simulink model "ctrl_TT_ad_ctrl_cpp_ros_feedback"  (R2022b)
settings: Solver=FixedStepAuto  StartTime=0.0  StopTime=Tf  FixedStep=0.05  RelTol=1e-3
StopFcn:
  | save('testdata')
values from neighbouring files (symbols this model uses):
  adap = 1    [testdata.mat]
  Ba_0 = [0 0 0 0 0 0]    [testdata.mat]
  Bb = 4418825.3321    [testdata.mat]
  Bv_0 = [-5.14444 0 0 0 0 0]    [testdata.mat]
  Bx_0 = [70.34790039 -18.70597267 -370.8000183 0 0 0]    [testdata.mat]
  Cp = [-70.34790039 18.70597267 -370.8000183 -33.25566673 18.72042656 -369.9571533 3.8263092 17.99342728 -368.5174255 40.77630615 14.78142262 -366.2670288 ... (183 elements, 3x61)]    [testdata.mat]    (also in tester.m = [Cpx'; Cpy'; Cpz'])
  Cp_prime = [4.4510680392 0.0017344668 0.1011438 4.44985762706 -0.08575700726 0.1715736104 4.43452754992 -0.37550053768 0.2668049284 4.4276356638 -0.45576590634 0.3213246444 ... (183 elements, 3x61)]    [testdata.mat]
  d = 250    [testdata.mat]
  dA_BP1 = [0.00388591051125 0.00354364911083 0.00553040741788 0.00502167988714 0.0078585088908 0.00748424955325 0.0119232766011 0.0109054787122 0.0168329706434 0.016985509009 0.0156802934897 0.014556760782 ... (616 elements, 616x1)]    [testdata.mat]
  dA_BP2 = [0.00388594063171 0.00354357191533 0.00553040491113 0.00502170939051 0.00785855989083 0.00748435285791 0.0119232653011 0.0109054419481 0.0168329955973 0.0169854794658 0.015680230324 0.0145567225609 ... (616 elements, 616x1)]    [testdata.mat]
  dA_Hull = [0.896301676511 0.898896720864 0.884294141897 0.886832830172 0.870887902011 0.873360353662 0.856223658523 0.858613244346 0.840314828191 0.842595287849 0.823129385532 0.8253007603 ... (2914 elements, 2914x1)]    [testdata.mat]
  dA_PH = [0.00917454029683 0.00917454029683 0.00646521761836 0.00644666811643 0.011728531678 0.0107683420972 0.0165186720105 0.0100399866209 0.0121147162203 0.00917369783051 0.00917369783051 0.00646462373197 ... (550 elements, 550x1)]    [testdata.mat]
  dA_Sail = [0.08073747293 0.0655437895785 0.0678199581962 0.211496702297 0.185444652254 0.10949647106 0.0763960001413 0.0735864235671 0.0440728222699 0.281106392154 0.32735958292 0.104041938486 ... (564 elements, 564x1)]    [testdata.mat]
  dA_SProot = [0.0225345452169 0.0247277274893 0.0225345452169 0.0480467976325 0.0166447079844 0.0410754287554 0.0247277274893 0.0480467976325 0.0468898715351 0.0839833312794 0.0166447079844 0.0255016718 ... (904 elements, 904x1)]    [testdata.mat]
  dA_X1a = [0.0149621011817 0.0166706156701 0.0341149781095 0.0355915100668 0.0512235531199 0.0489176133683 0.0604458424392 0.0503279152264 0.0577124835488 0.0401555322121 0.044833653096 0.0251568218541 ... (200 elements, 200x1)]    [testdata.mat]
  dA_X1b = [0.0149621011817 0.0166706156701 0.0341149781095 0.0355915100668 0.0512235531199 0.0489176133683 0.0604458424392 0.0503279152264 0.0577124835488 0.0401555322121 0.044833653096 0.0251568218541 ... (200 elements, 200x1)]    [testdata.mat]
  dA_X2a = [0.0149620639393 0.0166705502855 0.0341150948266 0.0355913495849 0.051223110376 0.0489180393921 0.0604458270347 0.0503275686692 0.0577128112225 0.0401556683139 0.0448334591683 0.0251566482124 ... (200 elements, 200x1)]    [testdata.mat]
  dA_X2b = [0.0149620639393 0.0166705502855 0.0341150948266 0.0355913495849 0.051223110376 0.0489180393921 0.0604458270347 0.0503275686692 0.0577128112225 0.0401556683139 0.0448334591683 0.0251566482124 ... (200 elements, 200x1)]    [testdata.mat]
  dA_X3a = [0.0149621011817 0.0166706156701 0.0341149781095 0.0355915100668 0.0512235531199 0.0489176133683 0.0604458424392 0.0503279152264 0.0577124835488 0.0401555322121 0.044833653096 0.0251568218541 ... (200 elements, 200x1)]    [testdata.mat]
  dA_X3b = [0.0149621011817 0.0166706156701 0.0341149781095 0.0355915100668 0.0512235531199 0.0489176133683 0.0604458424392 0.0503279152264 0.0577124835488 0.0401555322121 0.044833653096 0.0251568218541 ... (200 elements, 200x1)]    [testdata.mat]
  dA_X4a = [0.0149621011817 0.0166706156701 0.0341149781095 0.0355915100668 0.0512235531199 0.0489176133683 0.0604458424392 0.0503279152264 0.0577124835488 0.0401555322121 0.044833653096 0.0251568218541 ... (200 elements, 200x1)]    [testdata.mat]
  dA_X4b = [0.0149621011817 0.0166706156701 0.0341149781095 0.0355915100668 0.0512235531199 0.0489176133683 0.0604458424392 0.0503279152264 0.0577124835488 0.0401555322121 0.044833653096 0.0251568218541 ... (200 elements, 200x1)]    [testdata.mat]
  Ixx = 52300000    [testdata.mat]
  Ixy = 0    [testdata.mat]
  Ixz = 0    [testdata.mat]
  Iyy = 1375000000    [testdata.mat]
  Iyz = 0    [testdata.mat]
  Izz = 1367000000    [testdata.mat]
  Kp = 0.1    [testdata.mat]
  L1 =     [testdata.mat]
  Mb = 4418825.3321    [testdata.mat]
  n_BP1 = [-0.7747315 -0.03638153 -0.4095958 0 -0.1221389 0 -0.01670914 0 0.005209626 0 0.03404154 0 ... (1848 elements, 616x3)]    [testdata.mat]
  n_BP2 = [-0.774731517 -0.0363815315 -0.409595788 0 -0.122138903 0 -0.0167091396 0 0.00520962616 0 0.0340415388 0 ... (1848 elements, 616x3)]    [testdata.mat]
  n_Hull = [-3.334458e-05 -1.700098e-14 -3.354233e-05 -1.686235e-14 -3.289162e-05 -1.685701e-14 -3.291391e-05 -1.698144e-14 -3.338145e-05 -1.688959e-14 -3.29289e-05 -1.682536e-14 ... (8742 elements, 2914x3)]    [testdata.mat]
  n_PH = [0 0 0.01711651 0.01711627 0.2676807 0.2676804 0.7675173 0.7675174 0.9857236 0 0 0.01711456 ... (1650 elements, 550x3)]    [testdata.mat]
  n_Sail = [-0.05126832 -0.05168081 -0.0485872 -0.03288998 -0.03203588 -0.04435105 -0.04335441 -0.04419429 -0.05169604 0.01094904 0.01649325 -0.03825178 ... (1692 elements, 564x3)]    [testdata.mat]
  n_SProot = [-0.7837688 -0.7969784 -0.7837688 -0.79448 -0.280412 -0.3378876 -0.7969784 -0.79448 -0.7910827 -0.3483897 -0.280412 -0.2790298 ... (2712 elements, 904x3)]    [testdata.mat]
  n_X2a = [-0.283297986 -0.283136904 -0.283195704 -0.28313759 -0.2831586 -0.283137113 -0.28313911 -0.283136606 -0.283121586 -0.283136815 -0.283108413 -0.283138901 ... (600 elements, 200x3)]    [testdata.mat]
  n_X2b = [-0.283297986 -0.283136904 -0.283195704 -0.28313759 -0.2831586 -0.283137113 -0.28313911 -0.283136606 -0.283121586 -0.283136815 -0.283108413 -0.283138901 ... (600 elements, 200x3)]    [testdata.mat]
  n_X3a = [-0.283298 -0.2831369 -0.2831957 -0.2831376 -0.2831586 -0.2831371 -0.2831391 -0.2831366 -0.2831216 -0.2831368 -0.2831084 -0.2831389 ... (600 elements, 200x3)]    [testdata.mat]
  n_X4a = [-0.283298 -0.2831369 -0.2831957 -0.2831376 -0.2831586 -0.2831371 -0.2831391 -0.2831366 -0.2831216 -0.2831368 -0.2831084 -0.2831389 ... (600 elements, 200x3)]    [testdata.mat]
  n_X4b = [-0.283298 -0.2831369 -0.2831957 -0.2831376 -0.2831586 -0.2831371 -0.2831391 -0.2831366 -0.2831216 -0.2831368 -0.2831084 -0.2831389 ... (600 elements, 200x3)]    [testdata.mat]
  nt_BP1 = 616    [testdata.mat]
  nt_BP2 = 616    [testdata.mat]
  nt_Hull = 2914    [testdata.mat]
  nt_PH = 550    [testdata.mat]
  nt_Sail = 564    [testdata.mat]
  nt_SProot = 904    [testdata.mat]
  nt_X1a = 200    [testdata.mat]
  nt_X1b = 200    [testdata.mat]
  nt_X2a = 200    [testdata.mat]
  nt_X2b = 200    [testdata.mat]
  nt_X3a = 200    [testdata.mat]
  nt_X3b = 200    [testdata.mat]
  nt_X4a = 200    [testdata.mat]
  nt_X4b = 200    [testdata.mat]
  Seastate = 0    [testdata.mat]
  Tf = 500    [testdata.mat]    (also in tester.m)
  Ts = 0.05    [testdata.mat]
  vt1_BP1 = [-11.0524049722 -10.9924120522 -10.9924120522 -10.8819663922 -10.8819663922 -10.7297166322 -10.7297166322 -10.5070632922 -10.5070632922 -10.1807245522 -10.1807245522 -9.8815181122 ... (1848 elements, 616x3)]    [testdata.mat]
  vt1_BP2 = [-11.0524048318 -10.9924111396 -10.9924111396 -10.8819658306 -10.8819658306 -10.7297157898 -10.7297157898 -10.5070637134 -10.5070637134 -10.1807238502 -10.1807238502 -9.8815188844 ... (1848 elements, 616x3)]    [testdata.mat]
  vt1_Hull = [3.5122487678 3.7304022878 5.2621803278 5.4863499878 6.9866994878 7.2167238278 8.6832650078 8.9189474678 10.3493567078 10.5904445678 11.9823842078 12.2286247478 ... (8742 elements, 2914x3)]    [testdata.mat]
  vt1_PH = [37.3342788278 37.3342788278 37.4268866678 37.4268866678 37.5892452278 37.5892452278 37.7549453078 37.7549453078 37.8074619278 37.3342788278 37.3342788278 37.4268866678 ... (1650 elements, 550x3)]    [testdata.mat]
  vt1_Sail = [-12.4909433722 -12.1578443722 -12.0399645322 -11.2138368922 -10.6240515922 -11.5111900522 -11.9364967522 -11.6561249722 -12.4909433722 -7.5732648922 -6.8453119522 -11.1890071522 ... (1692 elements, 564x3)]    [testdata.mat]
  vt1_SProot = [29.2099766678 29.1371231078 29.0494854278 29.2099766678 29.2862630078 29.4526510478 29.0494854278 29.1261368078 29.3369263478 29.5706712878 29.0494854278 29.3857364078 ... (2712 elements, 904x3)]    [testdata.mat]
  vt1_X1a = [29.3961751478 29.4776282078 29.4776282078 29.7060309278 29.7060309278 30.0693861278 30.0693861278 30.5458756478 30.5458756478 31.0830460478 31.0830460478 31.6023926678 ... (600 elements, 200x3)]    [testdata.mat]
  vt1_X1b = [29.6638337078 29.6638337078 29.9620713878 29.9620713878 30.3181187678 30.3181187678 30.7116389078 30.7116389078 31.1104380878 31.1104380878 31.4810519678 31.4810519678 ... (600 elements, 200x3)]    [testdata.mat]
  vt1_X2a = [29.3961767624 29.4776272952 29.4776272952 29.7060326828 29.7060326828 30.0693842324 30.0693842324 30.5458736822 30.5458736822 31.083047171 31.083047171 31.6023916148 ... (600 elements, 200x3)]    [testdata.mat]
  vt1_X2b = [29.6638345502 29.6638345502 29.9620708964 29.9620708964 30.3181168022 30.3181168022 30.7116409436 30.7116409436 31.1104372454 31.1104372454 31.4810526698 31.4810526698 ... (600 elements, 200x3)]    [testdata.mat]
  vt1_X3a = [29.3961751478 29.4776282078 29.4776282078 29.7060309278 29.7060309278 30.0693861278 30.0693861278 30.5458756478 30.5458756478 31.0830460478 31.0830460478 31.6023926678 ... (600 elements, 200x3)]    [testdata.mat]
  vt1_X3b = [29.6638337078 29.6638337078 29.9620713878 29.9620713878 30.3181187678 30.3181187678 30.7116389078 30.7116389078 31.1104380878 31.1104380878 31.4810519678 31.4810519678 ... (600 elements, 200x3)]    [testdata.mat]
  vt1_X4a = [29.6638337078 29.6638337078 29.9620713878 29.9620713878 30.3181187678 30.3181187678 30.7116389078 30.7116389078 31.1104380878 31.1104380878 31.4810519678 31.4810519678 ... (600 elements, 200x3)]    [testdata.mat]
  vt1_X4b = [29.3961751478 29.4776282078 29.4776282078 29.7060309278 29.7060309278 30.0693861278 30.0693861278 30.5458756478 30.5458756478 31.0830460478 31.0830460478 31.6023926678 ... (600 elements, 200x3)]    [testdata.mat]
  vt2_BP1 = [-10.9924120522 -10.9494777322 -10.8819663922 -10.8505308322 -10.7297166322 -10.7112259522 -10.5070632922 -10.4997203722 -10.1807245522 -10.1757543922 -9.8815181122 -9.8813004922 ... (1848 elements, 616x3)]    [testdata.mat]
  vt2_BP2 = [-11.0294626294 -11.0294626294 -10.9494786448 -10.9494786448 -10.8505316746 -10.8505316746 -10.7112256012 -10.7112256012 -10.499720302 -10.499720302 -10.1757550942 -10.1757550942 ... (1848 elements, 616x3)]    [testdata.mat]
  vt2_Hull = [1.9517168078 1.9517168078 3.7304022878 3.7304022878 5.4863499878 5.4863499878 7.2167238278 7.2167238278 8.9189474678 8.9189474678 10.5904445678 10.5904445678 ... (8742 elements, 2914x3)]    [testdata.mat]
  vt2_PH = [37.2028433678 37.2028433678 37.3342788278 37.4268866678 37.4268866678 37.5892452278 37.5892452278 37.7549453078 37.7549453078 37.2028433678 37.2028433678 37.3342788278 ... (1650 elements, 550x3)]    [testdata.mat]
  vt2_Sail = [-12.0399645322 -12.0399645322 -11.9364967522 -10.7084881522 -10.7084881522 -12.0399645322 -12.0399645322 -11.9364967522 -12.3734566522 -7.7110323922 -7.7110323922 -11.6561249722 ... (1692 elements, 564x3)]    [testdata.mat]
  vt2_SProot = [29.0494854278 29.0494854278 29.2099766678 29.1261368078 29.0494854278 29.1371231078 29.1371231078 29.2099766678 29.1261368078 29.2099766678 29.2862630078 29.2862630078 ... (2712 elements, 904x3)]    [testdata.mat]
  vt2_X1a = [29.4776282078 29.9620713878 29.7060309278 30.3181187678 30.0693861278 30.7116389078 30.5458756478 31.1104380878 31.0830460478 31.4810519678 31.6023926678 31.7970362078 ... (600 elements, 200x3)]    [testdata.mat]
  vt2_X1b = [29.4776282078 29.9620713878 29.7060309278 30.3181187678 30.0693861278 30.7116389078 30.5458756478 31.1104380878 31.0830460478 31.4810519678 31.6023926678 31.7970362078 ... (600 elements, 200x3)]    [testdata.mat]
  vt2_X2a = [29.6638345502 29.6638345502 29.9620708964 29.9620708964 30.3181168022 30.3181168022 30.7116409436 30.7116409436 31.1104372454 31.1104372454 31.4810526698 31.4810526698 ... (600 elements, 200x3)]    [testdata.mat]
  vt2_X2b = [29.3961767624 29.4776272952 29.4776272952 29.7060326828 29.7060326828 30.0693842324 30.0693842324 30.5458736822 30.5458736822 31.083047171 31.083047171 31.6023916148 ... (600 elements, 200x3)]    [testdata.mat]
  vt2_X3a = [29.4776282078 29.9620713878 29.7060309278 30.3181187678 30.0693861278 30.7116389078 30.5458756478 31.1104380878 31.0830460478 31.4810519678 31.6023926678 31.7970362078 ... (600 elements, 200x3)]    [testdata.mat]
  vt2_X3b = [29.4776282078 29.9620713878 29.7060309278 30.3181187678 30.0693861278 30.7116389078 30.5458756478 31.1104380878 31.0830460478 31.4810519678 31.6023926678 31.7970362078 ... (600 elements, 200x3)]    [testdata.mat]
  vt2_X4a = [29.4776282078 29.9620713878 29.7060309278 30.3181187678 30.0693861278 30.7116389078 30.5458756478 31.1104380878 31.0830460478 31.4810519678 31.6023926678 31.7970362078 ... (600 elements, 200x3)]    [testdata.mat]
  vt2_X4b = [29.4776282078 29.9620713878 29.7060309278 30.3181187678 30.0693861278 30.7116389078 30.5458756478 31.1104380878 31.0830460478 31.4810519678 31.6023926678 31.7970362078 ... (600 elements, 200x3)]    [testdata.mat]
  vt3_BP1 = [-11.0294636122 -11.0294636122 -10.9494777322 -10.9494777322 -10.8505308322 -10.8505308322 -10.7112259522 -10.7112259522 -10.4997203722 -10.4997203722 -10.1757543922 -10.1757543922 ... (1848 elements, 616x3)]    [testdata.mat]
  vt3_BP2 = [-10.9924111396 -10.9494786448 -10.8819658306 -10.8505316746 -10.7297157898 -10.7112256012 -10.5070637134 -10.499720302 -10.1807238502 -10.1757550942 -9.8815188844 -9.8813013346 ... (1848 elements, 616x3)]    [testdata.mat]
  vt3_Hull = [1.7397198278 3.5122487678 3.5122487678 5.2621803278 5.2621803278 6.9866994878 6.9866994878 8.6832650078 8.6832650078 10.3493567078 10.3493567078 11.9823842078 ... (8742 elements, 2914x3)]    [testdata.mat]
  vt3_PH = [37.2028433678 37.3342788278 37.3342788278 37.3342788278 37.4268866678 37.4268866678 37.5892452278 37.5892452278 37.7549453078 37.2028433678 37.3342788278 37.3342788278 ... (1650 elements, 550x3)]    [testdata.mat]
  vt3_Sail = [-12.3734566522 -12.4909433722 -12.3734566522 -11.5111900522 -11.2138368922 -11.7698559922 -11.5111900522 -11.5111900522 -12.1578443722 -8.3109054322 -7.5732648922 -11.5111900522 ... (1692 elements, 564x3)]    [testdata.mat]
  vt3_SProot = [29.1261368078 29.2099766678 29.1261368078 29.3369263478 29.1371231078 29.2099766678 29.2099766678 29.3369263478 29.2548344678 29.3369263478 29.1371231078 29.1371231078 ... (2712 elements, 904x3)]    [testdata.mat]
  vt3_X1a = [29.6638337078 29.6638337078 29.9620713878 29.9620713878 30.3181187678 30.3181187678 30.7116389078 30.7116389078 31.1104380878 31.1104380878 31.4810519678 31.4810519678 ... (600 elements, 200x3)]    [testdata.mat]
  vt3_X1b = [29.3961751478 29.4776282078 29.4776282078 29.7060309278 29.7060309278 30.0693861278 30.0693861278 30.5458756478 30.5458756478 31.0830460478 31.0830460478 31.6023926678 ... (600 elements, 200x3)]    [testdata.mat]
  vt3_X2a = [29.4776272952 29.9620708964 29.7060326828 30.3181168022 30.0693842324 30.7116409436 30.5458736822 31.1104372454 31.083047171 31.4810526698 31.6023916148 31.7970343826 ... (600 elements, 200x3)]    [testdata.mat]
  vt3_X2b = [29.4776272952 29.9620708964 29.7060326828 30.3181168022 30.0693842324 30.7116409436 30.5458736822 31.1104372454 31.083047171 31.4810526698 31.6023916148 31.7970343826 ... (600 elements, 200x3)]    [testdata.mat]
  vt3_X3a = [29.6638337078 29.6638337078 29.9620713878 29.9620713878 30.3181187678 30.3181187678 30.7116389078 30.7116389078 31.1104380878 31.1104380878 31.4810519678 31.4810519678 ... (600 elements, 200x3)]    [testdata.mat]
  vt3_X3b = [29.3961751478 29.4776282078 29.4776282078 29.7060309278 29.7060309278 30.0693861278 30.0693861278 30.5458756478 30.5458756478 31.0830460478 31.0830460478 31.6023926678 ... (600 elements, 200x3)]    [testdata.mat]
  vt3_X4a = [29.3961751478 29.4776282078 29.4776282078 29.7060309278 29.7060309278 30.0693861278 30.0693861278 30.5458756478 30.5458756478 31.0830460478 31.0830460478 31.6023926678 ... (600 elements, 200x3)]    [testdata.mat]
  vt3_X4b = [29.6638337078 29.6638337078 29.9620713878 29.9620713878 30.3181187678 30.3181187678 30.7116389078 30.7116389078 31.1104380878 31.1104380878 31.4810519678 31.4810519678 ... (600 elements, 200x3)]    [testdata.mat]
  Xb = 0    [testdata.mat]
  Xcg = [32.3287332922 0 0]    [testdata.mat]
  Xg = 0    [testdata.mat]
  Yb = 0    [testdata.mat]
  Yg = 0    [testdata.mat]
  Zb = 0.4406    [testdata.mat]
  Zg = 0    [testdata.mat]
libraries: robotlib x54, simulink x8, sharedtransform x2, dspmathops x2
(part 5 of 9)

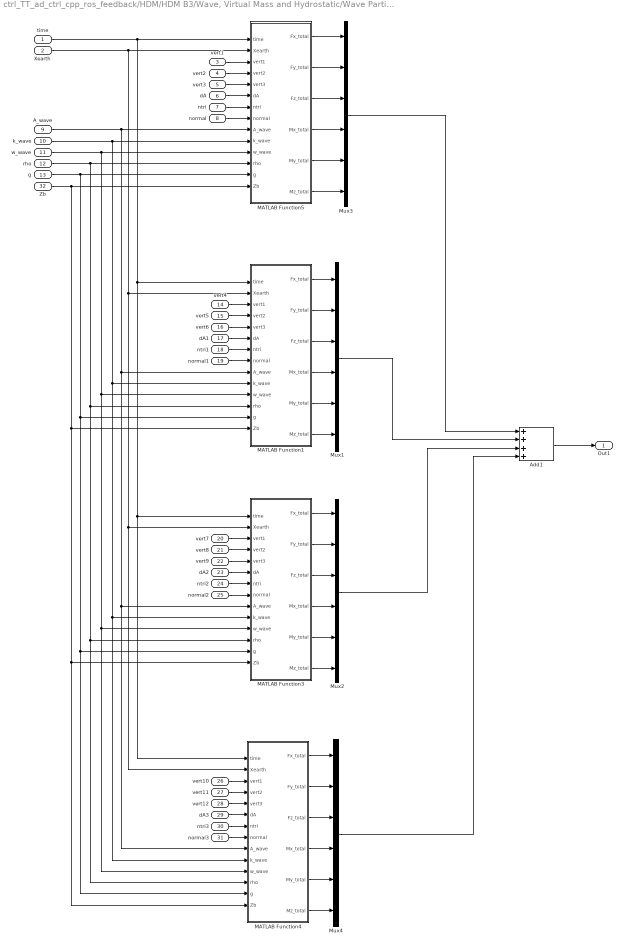
== system ctrl_TT_ad_ctrl_cpp_ros_feedback/HDM/HDM B3/Wave, Virtual Mass and Hydrostatic/Wave Particle Motions/Hydrostatic Forces and Moments/Subsystem ==
  time : Inport
  Xearth : Inport  Port=2
  vert1 : Inport  Port=3
  vert2 : Inport  Port=4
  vert3 : Inport  Port=5
  dA : Inport  Port=6
  ntri : Inport  Port=7
  normal : Inport  Port=8
  A_wave : Inport  Port=9
  k_wave : Inport  Port=10
  w_wave : Inport  Port=11
  rho : Inport  Port=12
  g : Inport  Port=13
  vert4 : Inport  Port=14
  vert5 : Inport  Port=15
  vert6 : Inport  Port=16
  dA1 : Inport  Port=17
  ntri1 : Inport  Port=18
  normal1 : Inport  Port=19
  vert7 : Inport  Port=20
  vert8 : Inport  Port=21
  vert9 : Inport  Port=22
  dA2 : Inport  Port=23
  ntri2 : Inport  Port=24
  normal2 : Inport  Port=25
  vert10 : Inport  Port=26
  vert11 : Inport  Port=27
  vert12 : Inport  Port=28
  dA3 : Inport  Port=29
  ntri3 : Inport  Port=30
  normal3 : Inport  Port=31
  Zb : Inport  Port=32
  Add1 : Sum  Inputs=4
  MATLAB Function1 : MATLAB Function  TreatAsAtomicUnit=on
  MATLAB Function3 : MATLAB Function  TreatAsAtomicUnit=on
  MATLAB Function4 : MATLAB Function  TreatAsAtomicUnit=on
  MATLAB Function5 : MATLAB Function  TreatAsAtomicUnit=on
  Mux{1..4} (4 alike) : Mux  Inputs=6
  Out1 : Outport
  wires:
  Mux4/1 -> Add1/4
  MATLAB Function4/5(My_total) -> Mux4/5
  MATLAB Function4/4(Mx_total) -> Mux4/4
  MATLAB Function4/3(Fz_total) -> Mux4/3
  MATLAB Function4/2(Fy_total) -> Mux4/2
  MATLAB Function4/1(Fx_total) -> Mux4/1
  MATLAB Function4/6(Mz_total) -> Mux4/6
  MATLAB Function3/6(Mz_total) -> Mux2/6
  MATLAB Function3/1(Fx_total) -> Mux2/1
  MATLAB Function3/2(Fy_total) -> Mux2/2
  MATLAB Function3/3(Fz_total) -> Mux2/3
  MATLAB Function3/4(Mx_total) -> Mux2/4
  MATLAB Function3/5(My_total) -> Mux2/5
  MATLAB Function1/5(My_total) -> Mux1/5
  MATLAB Function1/4(Mx_total) -> Mux1/4
  MATLAB Function1/3(Fz_total) -> Mux1/3
  MATLAB Function1/2(Fy_total) -> Mux1/2
  MATLAB Function1/1(Fx_total) -> Mux1/1
  Mux1/1 -> Add1/2
  MATLAB Function1/6(Mz_total) -> Mux1/6
  Mux2/1 -> Add1/3
  Zb/1 -> MATLAB Function4/14(Zb), MATLAB Function3/14(Zb), MATLAB Function1/14(Zb), MATLAB Function5/14(Zb)
  vert8/1 -> MATLAB Function3/4(vert2)
  vert1/1 -> MATLAB Function5/3(vert1)
  vert10/1 -> MATLAB Function4/3(vert1)
  dA1/1 -> MATLAB Function1/6(dA)
  normal2/1 -> MATLAB Function3/8(normal)
  vert3/1 -> MATLAB Function5/5(vert3)
  vert6/1 -> MATLAB Function1/5(vert3)
  Add1/1 -> Out1/1
  vert2/1 -> MATLAB Function5/4(vert2)
  dA3/1 -> MATLAB Function4/6(dA)
  ntri3/1 -> MATLAB Function4/7(ntri)
  ntri2/1 -> MATLAB Function3/7(ntri)
  vert11/1 -> MATLAB Function4/4(vert2)
  MATLAB Function5/6(Mz_total) -> Mux3/6
  dA/1 -> MATLAB Function5/6(dA)
  normal/1 -> MATLAB Function5/8(normal)
  vert9/1 -> MATLAB Function3/5(vert3)
  vert4/1 -> MATLAB Function1/3(vert1)
  normal3/1 -> MATLAB Function4/8(normal)
  vert12/1 -> MATLAB Function4/5(vert3)
  MATLAB Function5/1(Fx_total) -> Mux3/1
  dA2/1 -> MATLAB Function3/6(dA)
  g/1 -> MATLAB Function3/13(g), MATLAB Function4/13(g), MATLAB Function1/13(g), MATLAB Function5/13(g)
  ntri/1 -> MATLAB Function5/7(ntri)
  MATLAB Function5/2(Fy_total) -> Mux3/2
  w_wave/1 -> MATLAB Function3/11(w_wave), MATLAB Function4/11(w_wave), MATLAB Function1/11(w_wave), MATLAB Function5/11(w_wave)
  k_wave/1 -> MATLAB Function3/10(k_wave), MATLAB Function4/10(k_wave), MATLAB Function1/10(k_wave), MATLAB Function5/10(k_wave)
  MATLAB Function5/3(Fz_total) -> Mux3/3
  A_wave/1 -> MATLAB Function3/9(A_wave), MATLAB Function4/9(A_wave), MATLAB Function1/9(A_wave), MATLAB Function5/9(A_wave)
  normal1/1 -> MATLAB Function1/8(normal)
  Mux3/1 -> Add1/1
  MATLAB Function5/4(Mx_total) -> Mux3/4
  vert7/1 -> MATLAB Function3/3(vert1)
  Xearth/1 -> MATLAB Function1/2(Xearth), MATLAB Function3/2(Xearth), MATLAB Function4/2(Xearth), MATLAB Function5/2(Xearth)
  time/1 -> MATLAB Function3/1(time), MATLAB Function4/1(time), MATLAB Function1/1(time), MATLAB Function5/1(time)
  MATLAB Function5/5(My_total) -> Mux3/5
  vert5/1 -> MATLAB Function1/4(vert2)
  rho/1 -> MATLAB Function3/12(rho), MATLAB Function4/12(rho), MATLAB Function1/12(rho), MATLAB Function5/12(rho)
  ntri1/1 -> MATLAB Function1/7(ntri)

== system ctrl_TT_ad_ctrl_cpp_ros_feedback/HDM/HDM B3/Wave, Virtual Mass and Hydrostatic/Wave Particle Motions/Hydrostatic Forces and Moments/X1 ==
  time : Inport
  Xearth : Inport  Port=2
  vert1 : Inport  Port=3
  vert2 : Inport  Port=4
  vert3 : Inport  Port=5
  dA : Inport  Port=6
  ntri : Inport  Port=7
  A_wave : Inport  Port=8
  k_wave : Inport  Port=9
  w_wave : Inport  Port=10
  rho : Inport  Port=11
  g : Inport  Port=12
  vert4 : Inport  Port=13
  vert5 : Inport  Port=14
  vert6 : Inport  Port=15
  dA1 : Inport  Port=16
  ntri1 : Inport  Port=17
  Zb : Inport  Port=18
  EAX : Inport  Port=19
  dX : Inport  Port=20
  Root_o : Inport  Port=21
  Add1 : Sum
  CG : Constant  Value=[32.3114; 0; 0;]
  MATLAB Function1 : MATLAB Function  TreatAsAtomicUnit=on
  MATLAB Function4 : MATLAB Function  TreatAsAtomicUnit=on
  Mux1 : Mux  Inputs=6
  Mux2 : Mux  Inputs=6
  Out1 : Outport
  wires:
  MATLAB Function1/6(Mz_total) -> Mux1/6
  MATLAB Function1/5(My_total) -> Mux1/5
  CG/1 -> MATLAB Function4/17(xcg), MATLAB Function1/17(xcg)
  Root_o/1 -> MATLAB Function4/16(origin), MATLAB Function1/16(origin)
  dX/1 -> MATLAB Function1/15(dX), MATLAB Function4/15(dX)
  EAX/1 -> MATLAB Function4/14(EAX), MATLAB Function1/14(EAX)
  MATLAB Function4/3(Fz_total) -> Mux2/3
  MATLAB Function4/4(Mx_total) -> Mux2/4
  w_wave/1 -> MATLAB Function4/10(w_wave), MATLAB Function1/10(w_wave)
  MATLAB Function1/2(Fy_total) -> Mux1/2
  Xearth/1 -> MATLAB Function1/2(Xearth), MATLAB Function4/2(Xearth)
  rho/1 -> MATLAB Function4/11(rho), MATLAB Function1/11(rho)
  A_wave/1 -> MATLAB Function4/8(A_wave), MATLAB Function1/8(A_wave)
  MATLAB Function1/4(Mx_total) -> Mux1/4
  MATLAB Function4/1(Fx_total) -> Mux2/1
  MATLAB Function1/1(Fx_total) -> Mux1/1
  Add1/1 -> Out1/1
  MATLAB Function1/3(Fz_total) -> Mux1/3
  MATLAB Function4/5(My_total) -> Mux2/5
  dA/1 -> MATLAB Function4/6(dA)
  k_wave/1 -> MATLAB Function1/9(k_wave), MATLAB Function4/9(k_wave)
  g/1 -> MATLAB Function4/12(g), MATLAB Function1/12(g)
  MATLAB Function4/6(Mz_total) -> Mux2/6
  MATLAB Function4/2(Fy_total) -> Mux2/2
  Mux2/1 -> Add1/1
  vert3/1 -> MATLAB Function4/5(vert3)
  Mux1/1 -> Add1/2
  vert1/1 -> MATLAB Function4/3(vert1)
  time/1 -> MATLAB Function1/1(time), MATLAB Function4/1(time)
  ntri/1 -> MATLAB Function4/7(ntri)
  vert2/1 -> MATLAB Function4/4(vert2)
  Zb/1 -> MATLAB Function4/13(Zb), MATLAB Function1/13(Zb)
  vert4/1 -> MATLAB Function1/3(vert1)
  vert5/1 -> MATLAB Function1/4(vert2)
  vert6/1 -> MATLAB Function1/5(vert3)
  dA1/1 -> MATLAB Function1/6(dA)
  ntri1/1 -> MATLAB Function1/7(ntri)

== system ctrl_TT_ad_ctrl_cpp_ros_feedback/HDM/HDM B3/Wave, Virtual Mass and Hydrostatic/Wave Particle Motions/Hydrostatic Forces and Moments/X2 ==
  time : Inport
  Xearth : Inport  Port=2
  vert1 : Inport  Port=3
  vert2 : Inport  Port=4
  vert3 : Inport  Port=5
  dA : Inport  Port=6
  ntri : Inport  Port=7
  normal : Inport  Port=8
  A_wave : Inport  Port=9
  k_wave : Inport  Port=10
  w_wave : Inport  Port=11
  rho : Inport  Port=12
  g : Inport  Port=13
  vert4 : Inport  Port=14
  vert5 : Inport  Port=15
  vert6 : Inport  Port=16
  dA1 : Inport  Port=17
  ntri1 : Inport  Port=18
  Zb : Inport  Port=19
  EAX : Inport  Port=20
  dX : Inport  Port=21
  Root_o : Inport  Port=22
  Add1 : Sum
  CG : Constant  Value=[32.3114; 0; 0;]
  MATLAB Function1 : MATLAB Function  TreatAsAtomicUnit=on
  MATLAB Function4 : MATLAB Function  TreatAsAtomicUnit=on
  Mux1 : Mux  Inputs=6
  Mux2 : Mux  Inputs=6
  Out1 : Outport
  wires:
  ntri1/1 -> MATLAB Function1/7(ntri)
  dA1/1 -> MATLAB Function1/6(dA)
  vert6/1 -> MATLAB Function1/5(vert3)
  vert5/1 -> MATLAB Function1/4(vert2)
  vert4/1 -> MATLAB Function1/3(vert1)
  Zb/1 -> MATLAB Function4/13(Zb), MATLAB Function1/13(Zb)
  vert2/1 -> MATLAB Function4/4(vert2)
  ntri/1 -> MATLAB Function4/7(ntri)
  normal/1 -> ?
  time/1 -> MATLAB Function4/1(time), MATLAB Function1/1(time)
  vert1/1 -> MATLAB Function4/3(vert1)
  Mux1/1 -> Add1/2
  vert3/1 -> MATLAB Function4/5(vert3)
  Mux2/1 -> Add1/1
  MATLAB Function4/2(Fy_total) -> Mux2/2
  MATLAB Function4/6(Mz_total) -> Mux2/6
  g/1 -> MATLAB Function4/12(g), MATLAB Function1/12(g)
  k_wave/1 -> MATLAB Function4/9(k_wave), MATLAB Function1/9(k_wave)
  dA/1 -> MATLAB Function4/6(dA)
  MATLAB Function4/5(My_total) -> Mux2/5
  MATLAB Function1/3(Fz_total) -> Mux1/3
  Add1/1 -> Out1/1
  MATLAB Function1/1(Fx_total) -> Mux1/1
  MATLAB Function4/1(Fx_total) -> Mux2/1
  MATLAB Function1/4(Mx_total) -> Mux1/4
  A_wave/1 -> MATLAB Function4/8(A_wave), MATLAB Function1/8(A_wave)
  rho/1 -> MATLAB Function4/11(rho), MATLAB Function1/11(rho)
  Xearth/1 -> MATLAB Function4/2(Xearth), MATLAB Function1/2(Xearth)
  MATLAB Function1/2(Fy_total) -> Mux1/2
  w_wave/1 -> MATLAB Function4/10(w_wave), MATLAB Function1/10(w_wave)
  MATLAB Function4/4(Mx_total) -> Mux2/4
  MATLAB Function4/3(Fz_total) -> Mux2/3
  EAX/1 -> MATLAB Function4/14(EAX), MATLAB Function1/14(EAX)
  dX/1 -> MATLAB Function4/15(dX), MATLAB Function1/15(dX)
  Root_o/1 -> MATLAB Function4/16(origin), MATLAB Function1/16(origin)
  CG/1 -> MATLAB Function4/17(xcg), MATLAB Function1/17(xcg)
  MATLAB Function1/5(My_total) -> Mux1/5
  MATLAB Function1/6(Mz_total) -> Mux1/6

== system ctrl_TT_ad_ctrl_cpp_ros_feedback/HDM/HDM B3/Wave, Virtual Mass and Hydrostatic/Wave Particle Motions/Hydrostatic Forces and Moments/X3 ==
  time : Inport
  Xearth : Inport  Port=2
  vert1 : Inport  Port=3
  vert2 : Inport  Port=4
  vert3 : Inport  Port=5
  dA : Inport  Port=6
  ntri : Inport  Port=7
  A_wave : Inport  Port=8
  k_wave : Inport  Port=9
  w_wave : Inport  Port=10
  rho : Inport  Port=11
  g : Inport  Port=12
  vert4 : Inport  Port=13
  vert5 : Inport  Port=14
  vert6 : Inport  Port=15
  dA1 : Inport  Port=16
  ntri1 : Inport  Port=17
  Zb : Inport  Port=18
  EAX : Inport  Port=19
  dX : Inport  Port=20
  Root_o : Inport  Port=21
  Add1 : Sum
  CG : Constant  Value=[32.3114; 0; 0;]
  MATLAB Function1 : MATLAB Function  TreatAsAtomicUnit=on
  MATLAB Function4 : MATLAB Function  TreatAsAtomicUnit=on
  Mux1 : Mux  Inputs=6
  Mux2 : Mux  Inputs=6
  Out1 : Outport
  wires:
  MATLAB Function1/6(Mz_total) -> Mux1/6
  MATLAB Function1/5(My_total) -> Mux1/5
  CG/1 -> MATLAB Function1/17(xcg), MATLAB Function4/17(xcg)
  Root_o/1 -> MATLAB Function1/16(origin), MATLAB Function4/16(origin)
  dX/1 -> MATLAB Function1/15(dX), MATLAB Function4/15(dX)
  EAX/1 -> MATLAB Function1/14(EAX), MATLAB Function4/14(EAX)
  MATLAB Function4/3(Fz_total) -> Mux2/3
  MATLAB Function4/4(Mx_total) -> Mux2/4
  w_wave/1 -> MATLAB Function1/10(w_wave), MATLAB Function4/10(w_wave)
  MATLAB Function1/2(Fy_total) -> Mux1/2
  Xearth/1 -> MATLAB Function1/2(Xearth), MATLAB Function4/2(Xearth)
  rho/1 -> MATLAB Function1/11(rho), MATLAB Function4/11(rho)
  A_wave/1 -> MATLAB Function1/8(A_wave), MATLAB Function4/8(A_wave)
  MATLAB Function1/4(Mx_total) -> Mux1/4
  MATLAB Function4/1(Fx_total) -> Mux2/1
  MATLAB Function1/1(Fx_total) -> Mux1/1
  Add1/1 -> Out1/1
  MATLAB Function1/3(Fz_total) -> Mux1/3
  MATLAB Function4/5(My_total) -> Mux2/5
  dA/1 -> MATLAB Function4/6(dA)
  k_wave/1 -> MATLAB Function1/9(k_wave), MATLAB Function4/9(k_wave)
  g/1 -> MATLAB Function1/12(g), MATLAB Function4/12(g)
  MATLAB Function4/6(Mz_total) -> Mux2/6
  MATLAB Function4/2(Fy_total) -> Mux2/2
  Mux2/1 -> Add1/1
  vert3/1 -> MATLAB Function4/5(vert3)
  Mux1/1 -> Add1/2
  vert1/1 -> MATLAB Function4/3(vert1)
  time/1 -> MATLAB Function1/1(time), MATLAB Function4/1(time)
  ntri/1 -> MATLAB Function4/7(ntri)
  vert2/1 -> MATLAB Function4/4(vert2)
  Zb/1 -> MATLAB Function1/13(Zb), MATLAB Function4/13(Zb)
  vert4/1 -> MATLAB Function1/3(vert1)
  vert5/1 -> MATLAB Function1/4(vert2)
  vert6/1 -> MATLAB Function1/5(vert3)
  dA1/1 -> MATLAB Function1/6(dA)
  ntri1/1 -> MATLAB Function1/7(ntri)

== system ctrl_TT_ad_ctrl_cpp_ros_feedback/HDM/HDM B3/Wave, Virtual Mass and Hydrostatic/Wave Particle Motions/Hydrostatic Forces and Moments/X4 ==
  time : Inport
  Xearth : Inport  Port=2
  vert1 : Inport  Port=3
  vert2 : Inport  Port=4
  vert3 : Inport  Port=5
  dA : Inport  Port=6
  ntri : Inport  Port=7
  normal : Inport  Port=8
  A_wave : Inport  Port=9
  k_wave : Inport  Port=10
  w_wave : Inport  Port=11
  rho : Inport  Port=12
  g : Inport  Port=13
  vert4 : Inport  Port=14
  vert5 : Inport  Port=15
  vert6 : Inport  Port=16
  dA1 : Inport  Port=17
  ntri1 : Inport  Port=18
  Zb : Inport  Port=19
  EAX : Inport  Port=20
  dX : Inport  Port=21
  Root_o : Inport  Port=22
  Add1 : Sum
  CG : Constant  Value=[32.3114; 0; 0;]
  MATLAB Function1 : MATLAB Function  TreatAsAtomicUnit=on
  MATLAB Function4 : MATLAB Function  TreatAsAtomicUnit=on
  Mux1 : Mux  Inputs=6
  Mux2 : Mux  Inputs=6
  Out1 : Outport
  wires:
  ntri1/1 -> MATLAB Function1/7(ntri)
  dA1/1 -> MATLAB Function1/6(dA)
  vert6/1 -> MATLAB Function1/5(vert3)
  vert5/1 -> MATLAB Function1/4(vert2)
  vert4/1 -> MATLAB Function1/3(vert1)
  Zb/1 -> MATLAB Function4/13(Zb), MATLAB Function1/13(Zb)
  vert2/1 -> MATLAB Function4/4(vert2)
  ntri/1 -> MATLAB Function4/7(ntri)
  normal/1 -> ?
  time/1 -> MATLAB Function4/1(time), MATLAB Function1/1(time)
  vert1/1 -> MATLAB Function4/3(vert1)
  Mux1/1 -> Add1/2
  vert3/1 -> MATLAB Function4/5(vert3)
  Mux2/1 -> Add1/1
  MATLAB Function4/2(Fy_total) -> Mux2/2
  MATLAB Function4/6(Mz_total) -> Mux2/6
  g/1 -> MATLAB Function4/12(g), MATLAB Function1/12(g)
  k_wave/1 -> MATLAB Function4/9(k_wave), MATLAB Function1/9(k_wave)
  dA/1 -> MATLAB Function4/6(dA)
  MATLAB Function4/5(My_total) -> Mux2/5
  MATLAB Function1/3(Fz_total) -> Mux1/3
  Add1/1 -> Out1/1
  MATLAB Function1/1(Fx_total) -> Mux1/1
  MATLAB Function4/1(Fx_total) -> Mux2/1
  MATLAB Function1/4(Mx_total) -> Mux1/4
  A_wave/1 -> MATLAB Function4/8(A_wave), MATLAB Function1/8(A_wave)
  rho/1 -> MATLAB Function1/11(rho), MATLAB Function4/11(rho)
  Xearth/1 -> MATLAB Function4/2(Xearth), MATLAB Function1/2(Xearth)
  MATLAB Function1/2(Fy_total) -> Mux1/2
  w_wave/1 -> MATLAB Function4/10(w_wave), MATLAB Function1/10(w_wave)
  MATLAB Function4/4(Mx_total) -> Mux2/4
  MATLAB Function4/3(Fz_total) -> Mux2/3
  EAX/1 -> MATLAB Function4/14(EAX), MATLAB Function1/14(EAX)
  dX/1 -> MATLAB Function4/15(dX), MATLAB Function1/15(dX)
  Root_o/1 -> MATLAB Function4/16(origin), MATLAB Function1/16(origin)
  CG/1 -> MATLAB Function4/17(xcg), MATLAB Function1/17(xcg)
  MATLAB Function1/5(My_total) -> Mux1/5
  MATLAB Function1/6(Mz_total) -> Mux1/6

== system ctrl_TT_ad_ctrl_cpp_ros_feedback/HDM/HDM B3/Wave, Virtual Mass and Hydrostatic/Wave Particle Motions/Hydrostatic Forces and Moments/XB ==
  time : Inport
  Xearth : Inport  Port=2
  vert1 : Inport  Port=3
  vert2 : Inport  Port=4
  vert3 : Inport  Port=5
  dA : Inport  Port=6
  ntri : Inport  Port=7
  normal : Inport  Port=8
  A_wave : Inport  Port=9
  k_wave : Inport  Port=10
  w_wave : Inport  Port=11
  rho : Inport  Port=12
  g : Inport  Port=13
  vert4 : Inport  Port=14
  vert5 : Inport  Port=15
  vert6 : Inport  Port=16
  dA1 : Inport  Port=17
  ntri1 : Inport  Port=18
  normal1 : Inport  Port=19
  Zb : Inport  Port=20
  EAX : Inport  Port=21
  dX : Inport  Port=22
  Root_o : Inport  Port=23
  Add1 : Sum
  CG : Constant  Value=[32.3114; 0; 0;]
  MATLAB Function1 : MATLAB Function  TreatAsAtomicUnit=on
  MATLAB Function4 : MATLAB Function  TreatAsAtomicUnit=on
  Mux1 : Mux  Inputs=6
  Mux2 : Mux  Inputs=6
  Out1 : Outport
  wires:
  normal1/1 -> ?
  ntri1/1 -> MATLAB Function1/7(ntri)
  dA1/1 -> MATLAB Function1/6(dA)
  vert6/1 -> MATLAB Function1/5(vert3)
  vert5/1 -> MATLAB Function1/4(vert2)
  vert4/1 -> MATLAB Function1/3(vert1)
  Zb/1 -> MATLAB Function4/13(Zb), MATLAB Function1/13(Zb)
  vert2/1 -> MATLAB Function4/4(vert2)
  ntri/1 -> MATLAB Function4/7(ntri)
  normal/1 -> ?
  time/1 -> MATLAB Function4/1(time), MATLAB Function1/1(time)
  vert1/1 -> MATLAB Function4/3(vert1)
  Mux1/1 -> Add1/2
  vert3/1 -> MATLAB Function4/5(vert3)
  Mux2/1 -> Add1/1
  MATLAB Function4/2(Fy_total) -> Mux2/2
  MATLAB Function4/6(Mz_total) -> Mux2/6
  g/1 -> MATLAB Function4/12(g), MATLAB Function1/12(g)
  k_wave/1 -> MATLAB Function4/9(k_wave), MATLAB Function1/9(k_wave)
  dA/1 -> MATLAB Function4/6(dA)
  MATLAB Function4/5(My_total) -> Mux2/5
  MATLAB Function1/3(Fz_total) -> Mux1/3
  Add1/1 -> Out1/1
  MATLAB Function1/1(Fx_total) -> Mux1/1
  MATLAB Function4/1(Fx_total) -> Mux2/1
  MATLAB Function1/4(Mx_total) -> Mux1/4
  A_wave/1 -> MATLAB Function4/8(A_wave), MATLAB Function1/8(A_wave)
  rho/1 -> MATLAB Function4/11(rho), MATLAB Function1/11(rho)
  Xearth/1 -> MATLAB Function4/2(Xearth), MATLAB Function1/2(Xearth)
  MATLAB Function1/2(Fy_total) -> Mux1/2
  w_wave/1 -> MATLAB Function4/10(w_wave), MATLAB Function1/10(w_wave)
  MATLAB Function4/4(Mx_total) -> Mux2/4
  MATLAB Function4/3(Fz_total) -> Mux2/3
  EAX/1 -> MATLAB Function4/14(EAX), MATLAB Function1/14(EAX)
  dX/1 -> MATLAB Function4/15(dX), MATLAB Function1/15(dX)
  Root_o/1 -> MATLAB Function4/16(origin), MATLAB Function1/16(origin)
  CG/1 -> MATLAB Function4/17(xcg), MATLAB Function1/17(xcg)
  MATLAB Function1/5(My_total) -> Mux1/5
  MATLAB Function1/6(Mz_total) -> Mux1/6

== matlab function ctrl_TT_ad_ctrl_cpp_ros_feedback/Controller/Subsystem1/MATLAB Function ==
  data: u input; y output
function y = R3(u)

y = [u(1,1) u(1,2) 0; u(2,1) u(2,2) 0; 0 0 1];

== matlab function ctrl_TT_ad_ctrl_cpp_ros_feedback/Controller/MATLAB Function2 ==
  data: time input; pd output; pdp output; Cp_prime parameter; Cp parameter; Tf parameter
function [pd, pdp] = fcn(time, Cp_prime, Cp, Tf)




pd = BernsteinPoly(Cp,time,0,Tf);
pdp = BernsteinPoly(Cp_prime,time,0,Tf);

% pd = [gamma; gamma/2 ; -50];
% 
% 
% pdp = [1 ; 1/2; 0];

end










function  poly_t  = BernsteinPoly(Cp,t,t0,tf)

% INPUTS:
% Cp is a matrix n by N+1 (n: dimension of polynomial, N: order of polynomial) 
% t is a time vector
% OUTPUT:
% poly_t: n-dimensional polynomial evaluated at each time t

% if t is a scalar, it returns the value of Bernstein Poly at t in [t0,tf]
% if t0 and tf are not provided, it returns the value of Bernstein Poly at t in [0,1]

% Written by: Venanzio Cichella       

%%%%%%%%%%%%%%%%%%%%%%%%%%%%%%%%%%%%%%%%%%%%%%

coder.extrinsic('exist')

[~, N] = size(Cp);
N = N-1;


% if length(t) > 1
%     B = BernsteinMatrix_a2b(N,t)';
%     poly_t = Cp*B;
% else
%     if ~exist('t0','var')
%         B = BernsteinMatrix_a2b(N,t)';
%         poly_t = Cp*B;
%     else
%         B = BernsteinMatrix_a2b(N,t,t0,tf)';
%         poly_t = Cp*B;
%     end
% end
B = BernsteinMatrix_a2b(N,t,t0,tf)';
poly_t = Cp*B;


end










function b = BernsteinMatrix_a2b(N, t, tmin, tmax)

% Inputs: order N, time vector t = [t0 ... tm], no need for tmin and tmax.
% Output: b = [b0N(t0) b1N(t0) ... bNN(t0);
%              b0N(t1) b1N(t1) ... bNN(t1);
%              ...
%              b0N(tm) b1N(tm) ... bNN(tm);
% Use: If Cp is a row vector of N+1 control points,
%       the Nth order Bezier curve is given by xN=Cp*b';
% This function is used in BernsteinPoly

% Alternatively
% Inputs: order n, scalar time t', tmin and tmax
% Output: b = [b0n(t') b1n(t') ... bnn(t')]
% Use: If Cp is a row vector of N+1 control points,
%       the Nth order Bezier curve evaluated at t' is given by xn=Cp*b';
% Comment: This is more efficient but not as robust as de Casteljau
%           It works best for low-order curves

% Written by: Venanzio Cichella       

%%%%%%%%%%%%%%%%%%%%%%%%%%%%%%%%%%%%%%%%%%%%%%

if length(t) > 1
    tmax = t(length(t));
    tmin = t(1);
end
%coder.extrinsic('exist')
%if ~exist('tmin','var')
%    tmin = 0; tmax = 1;
%end



% compute B(j+1) = binomial(n, j), j = 0..n
t = t';
B = ones(N+1, 1); 
for j = 1:ceil(N/2)
  B(j+1) = B(j)*(N+1-j)/j;
  B(N+1-j) = B(j+1);
end
% compute T(i, j) = (t(i)-tmin)^j, TT(i, j) = (tmax-t(i))^(N-j)
T = ones(length(t), N+1);
TT = ones(length(t), N+1);
% turn a row t into a column t so that 
% we can do diag(t)*T(:,j) by t.*T(:,j)
tp = reshape(t, length(t), 1)-tmin;
ttp = tmax - t;
% Compute binomial(N, j)*(t(i)-tmin)^j*(tmax-t(i))^(N-j)
for j = 1:N 
  T(:, j+1) = tp .* T(:, j); 
  T(:, j) = T(:, j) .* B(j);
 TT(:,N+1-j) = ttp .* TT(:,N+2-j);
end

% Compute binomial(N, j)*(t(i)-tmin)^j*(tmax-t(i))^(N-j)/((tmax-tmin)^N)
b =  T.*TT./((tmax-tmin)^N);

end

== matlab function ctrl_TT_ad_ctrl_cpp_ros_feedback/Controller/Subsystem1/Subsystem2/MATLAB Function ==
  data: a input; y output; b input
function y = fcn(a,b)

%y = [a,b,0;-b,a,0;0,0,1];
y = [a,b;-b,a];

== matlab function ctrl_TT_ad_ctrl_cpp_ros_feedback/Controller/Marin PID ==
  settings: updateMethod=DISCRETE
  data: z_ref input; psi_ref input; Bv input; Bx input; dX output; Ts parameter
function dX   = fcn(z_ref,psi_ref,Bv,Bx,Ts)

persistent zerr_prev zerr_int_prev thetaerr_prev thetaerr_int_prev psierr_prev psierr_int_prev

%% Initialize
if isempty(zerr_prev)
        zerr_prev = 0;
        zerr_int_prev = 0;
        thetaerr_prev = 0;
        thetaerr_int_prev = 0;
        psierr_prev = 0;
        psierr_int_prev = 0;
end


%% Variables for feedback
x = Bx(1); y = Bx(2); z = Bx(3); phi = Bx(4); theta = Bx(5); psi = Bx(6);
p = [x;y;z];
uN = Bv(1); vN = Bv(2); wN = Bv(3); pB = Bv(4); qB=Bv(5); rB = Bv(6);
uB = -uN; vB = -vN; wB = wN;


%% Gains
KP_APz = 3;
KI_APz = 0*0.1044;
KD_APz = 3;

KP_APtheta = 3;
KI_APtheta = 0*0.1466;
KD_APtheta = 3;

KP_APpsi = 3;
KI_APpsi = 0;
KD_APpsi = 12.199;








%% Autopilot (depth)
zerr = z_ref - z;
zerrint = zerr*Ts+zerr_int_prev;
zerrdot = (zerr-zerr_prev)/Ts;
dvz = KP_APz*zerr+KI_APz*zerrint+KD_APz*zerrdot;

theta_ref = 0;
thetaerr = (theta_ref - theta)*180/pi;
thetaerrint = thetaerr*Ts+thetaerr_int_prev;
thetaerrdot = (thetaerr-thetaerr_prev)/Ts;
dvtheta = KP_APtheta*thetaerr+KI_APtheta*thetaerrint+KD_APtheta*thetaerrdot;

dv = dvz + dvtheta;

%% Autopilot (yaw)
psierr = (psi_ref - psi)*180/pi;
psierrint = psierr*Ts+psierr_int_prev;
psierrdot = (psierr-psierr_prev)/Ts;
dh = KP_APpsi*psierr+KI_APpsi*psierrint+KD_APpsi*psierrdot;


%% Control Allocation
d1 = -dv+dh; 
d2 = -dv-dh; 
d3 = dv-dh; 
d4 = dv+dh; 
d5 = dv; 
dX = [d1 ; d2 ; d3 ; d4 ; d5];





%% Save variables for next loop
zerr_prev = zerr;
zerr_int_prev = zerrint;
thetaerr_prev = thetaerr;
thetaerr_int_prev = thetaerrint;
psierr_prev = psierr;
psierr_int_prev = psierrint;

== matlab function ctrl_TT_ad_ctrl_cpp_ros_feedback/Controller/FF velocity ctrl ==
  settings: updateMethod=DISCRETE
  data: v_ref input; n output
function n   = fcn(v_ref)




KP_n = 5;
FF_inv = 4;



%% Prop
n = v_ref/FF_inv;

== matlab function ctrl_TT_ad_ctrl_cpp_ros_feedback/Controller/l1 aug - heading ==
  settings: updateMethod=DISCRETE
  data: y_ref input; Bv input; Bx input; y_aug output; Ts parameter; adap parameter; L1 parameter
function y_aug    = fcn(y_ref,Bv,Bx,Ts,adap,L1)
%pd,NomegaNI,

persistent xu xd


%% Variables for feedback
x = Bx(1); y = Bx(2); z = Bx(3); phi = Bx(4); theta = Bx(5); psi = Bx(6);
p = [x;y;z];
uN = Bv(1); vN = Bv(2); wN = Bv(3); pB = Bv(4); qB=Bv(5); rB = Bv(6);
uB = -uN; vB = -vN; wB = wN;

%% Control Parameters  
% Gains for PF augmentation
Ts = Ts;
Am = L1.Amz; Bm = L1.Bmz; Cm = L1.Cmz; 
Phiinv = L1.Phiinvz; Lambda = L1.Lambdaz;
Ao = L1.Aoz; Bo = L1.Boz; Co = L1.Coz;

%% Output Definition
y = psi;;

%% Initialize
if isempty(xu)
        xu = zeros(length(Ao),1);
        xd = Cm'*inv(Cm*Cm')*y;
        xu_next = xu;
        xd_next = xd;
end



%% L1 Augmentation - dive

if adap 

    yd = Cm*xd;
    vec1    =   [eye(size(Bm,2)); zeros(size(Am,1)-size(Bm,2),size(Bm,2))];
    sigma = -Phiinv*expm(Lambda*(Am/Lambda)*Ts)*vec1*(yd-y);

    xu_next = expm(Ao*Ts)*xu + inv(Ao)*(expm(Ao*Ts)-eye(length(Bo)))*(Bo*expm(-Am*Ts)*sigma);
    Kg = -inv(Cm*inv(Am)*Bm);
    ud = Kg*y_ref - Co*xu;

    xd_next = expm(Am*Ts)*xd + inv(Am)*(expm(Am*Ts)-eye(length(Am)))*(Bm*ud + sigma);

    y_aug = ud;

else 

    y_aug = y_ref;

    xd_next = xd;
    xu_next = xu;

end




%% Save variables for next loop
xu = xu_next;
xd = xd_next;

== matlab function ctrl_TT_ad_ctrl_cpp_ros_feedback/HDM/HDM B3/Effective Veloicity Calclation/MATLAB Function ==
  data: nh input; n1 input; aX output; n2 input; n3 input; n4 input; nB input; urX1 input; urX2 input; urX3 input; urX4 input; urXB input; UeX output
function [aX,UeX] = fcn(nh,n1,n2,n3,n4,nB,urX1,urX2,urX3,urX4,urXB)

%urXi: relative velocity of rigid body motion and wave particle velocity to the ith stern plane
%ni  : base vector of i-th plane's axis direction
%nh  : base vector of the hull axis direction
IP=zeros(5,1); %IP determines the sign of the angle of attack. if the dot product is negative, angle is greater than 90degs.
aX=zeros(5,1);

np1=dot(nh,urX1)*nh+dot(n1,urX1)*n1;
np2=dot(nh,urX2)*nh+dot(n2,urX2)*n2;
np3=dot(nh,urX3)*nh+dot(n3,urX3)*n3;
np4=dot(nh,urX4)*nh+dot(n4,urX4)*n4;
npB=dot(nh,urXB)*nh+dot(nB,urXB)*nB;

arg1=dot(np1,urX1)/(norm(np1)*norm(urX1));
arg2=dot(np2,urX2)/(norm(np2)*norm(urX2));
arg3=dot(np3,urX3)/(norm(np3)*norm(urX3));
arg4=dot(np4,urX4)/(norm(np4)*norm(urX4));
arg5=dot(npB,urXB)/(norm(npB)*norm(urXB));

%to prevent numerical error: acos returns complex solution. used if statement
if arg1 >=1
   aX(1,1)=0;
else
   aX(1,1)=acos(arg1)*180/pi*sqrt(2);
end

if arg2 >=1
   aX(2,1)=0;
else
   aX(2,1)=acos(arg2)*180/pi*sqrt(2);
end

if arg3 >=1
   aX(3,1)=0;
else
   aX(3,1)=acos(arg3)*180/pi*sqrt(2);
end

if arg4 >=1
   aX(4,1)=0;
else
   aX(4,1)=acos(arg4)*180/pi*sqrt(2);
end

if arg5 >=1
   aX(5,1)=0;
else
   aX(5,1)=acos(arg5)*180/pi;
end

d1=cross(n1,nh);
d2=cross(n2,nh);
d3=cross(n3,nh);
d4=cross(n4,nh);
dB=cross(nB,nh);

IP(1,1)=dot(d1,urX1);
IP(2,1)=dot(d2,urX2);
IP(3,1)=dot(d3,urX3);
IP(4,1)=dot(d4,urX4);
IP(5,1)=dot(dB,urXB);

for i=1:5
    if IP(i,1)<0
        aX(i,1)=-aX(i,1)
    end
end    

UeX=[norm(urX1); norm(urX2); norm(urX3); norm(urX4); norm(urXB);];
end

== matlab function ctrl_TT_ad_ctrl_cpp_ros_feedback/HDM/HDM B3/Effective Veloicity Calclation/MATLAB Function1 ==
  data: rX1 input; urX1 output; rX2 input; urX2 output; urX3 output; urX4 output; urXB output; rX3 input; rX4 input; rXB input; U_ship input
function [urX1,urX2,urX3,urX4,urXB]= fcn(rX1,rX2,rX3,rX4,rXB,U_ship)

%rXi: position vector of Stern planes from the CG
%rXB: position vector of sail planes from the CG
%U_ship: rigid body velcity in the ship system

u_ship=[U_ship(1); U_ship(2); U_ship(3);]
w_ship=[U_ship(4); U_ship(5); U_ship(6);]

urX1=-u_ship+cross(rX1,w_ship);
urX2=-u_ship+cross(rX2,w_ship);
urX3=-u_ship+cross(rX3,w_ship);
urX4=-u_ship+cross(rX4,w_ship);
urXB=-u_ship+cross(rXB,w_ship);

end

== matlab function ctrl_TT_ad_ctrl_cpp_ros_feedback/HDM/HDM B3/Effective Veloicity Calclation/MATLAB Function2 ==
  data: Bv input; alpha output; beta output; Umag output; uCG input; vCG input; wCG input
function [alpha,beta,Umag] = fcn(Bv,uCG,vCG,wCG)

    u_eff=uCG-Bv(1);
    v_eff=vCG-Bv(2);
    w_eff=wCG-Bv(3);
    
    U_eff=[u_eff; v_eff; w_eff;];
    
    if abs(u_eff) <= 1e-8
        alpha=90; beta=90;
        if v_eff < 0
            beta = -90;
        end
        if w_eff < 0
            alpha = -90;
        end
    else
        beta  = -atan(v_eff/u_eff)*180/pi;
        alpha =  atan(w_eff/u_eff)*180/pi;
    end
    
    Umag =norm(U_eff);
end

== matlab function ctrl_TT_ad_ctrl_cpp_ros_feedback/HDM/HDM B3/K/Mx ==
  data: Bx input; Bv input; Ba input; CKup input; CKur input; CKpp input; CKuvw input; Umag input; UeX input; dLCG input; dmass input; CNdXi input; K output; KApp output; K_hull output; Xg parameter; Bb parameter; Xb parameter; Mb parameter; Zg parameter; Zb parameter; Kh_total output; Kpp output; Kprop output; Kvm input; KAppAll output; BFK input; KStat output; Qprop input
function [K,KApp,K_hull,Kh_total,Kpp,Kprop,KAppAll,KStat]  = fcn(Bx,Bv,Ba, CKup,CKur,CKpp,CKuvw,Umag,UeX,dLCG,dmass,CNdXi,Xg,Bb,Xb,Mb,Zg,Zb,Kvm,BFK,Qprop)
%Bx,Bv,Ba are the body motion position, velocity, acceleration in ship coordinate
%Wv,Wa are the wave particle velocity, acceleration in ship coordinate

u=Bv(1); v=Bv(2); w=Bv(3); p=Bv(4); q=Bv(5); r=Bv(6);
x=Bx(1); y=Bx(2); z=Bx(3); phi=Bx(4); theta=Bx(5); psi=Bx(6);
a1=Ba(1); a2=Ba(2); a3=Ba(3); a4=Ba(4); a5=Ba(5); a6=Ba(6); 

KdX1=70.2^3*1025*CNdXi(1)*UeX(1)^2;
KdX2=70.2^3*1025*CNdXi(2)*UeX(2)^2;
KdX3=70.2^3*1025*CNdXi(3)*UeX(3)^2;
KdX4=70.2^3*1025*CNdXi(4)*UeX(4)^2;

Kup = -70.2^3*1025*(-2.9648E-04*u*p)*u^2;
Kur = 70.2^3*1025*(-5.6192E-05*u*r)*u^2;
Kpp = 70.2^3*1025*(-1.0622E-01*p*abs(p));
Kuvw=0.5*70.2^3*1025*CKuvw*Umag^2;
Kprop=Qprop;

KAppAll=[KdX1; KdX2; KdX3; KdX4;];

K_hull=Kuvw+Kup+Kur+Kpp;
KApp=KdX1+KdX2+KdX3+KdX4;
KStat= (Xg*(Mb+dmass))*cos(theta)*sin(phi)+BFK;%(Xg*(Mb+dmass)-Xb*Bb)*cos(theta)*sin(phi);
Kh_total=K_hull+KApp+KStat+Kpp+Kprop;
K=K_hull+KApp+KStat+Kvm+Kpp+Kprop;
end

== matlab function ctrl_TT_ad_ctrl_cpp_ros_feedback/HDM/HDM B3/M/My ==
  data: Bx input; Bv input; Ba input; Mqq input; Mwq input; Mprop input; Muvw input; Umag input; UeSP input; dLCG input; dmass input; MdXi input size=5; MY output; Xg parameter; Bb parameter; Xb parameter; Mb parameter; Zg parameter; Zb parameter; Mvm input; MYApp output; MYStat output; Mprop output; M_hull output; MY_hyd output; MYApp_All output; BFM input
function [MY, MYApp, MYStat, Mprop, M_hull,MY_hyd,MYApp_All] = fcn(Bx,Bv,Ba,Mqq,Mwq,Mprop,Muvw,Umag,UeSP,dLCG,dmass,MdXi,Xg,Bb,Xb,Mb,Zg,Zb,Mvm,BFM)
%wqfunction [MY,MYApp,MYStat,Mprop,M_hull]  = fcn(Bx,Bv,Ba,Mqq,Mwq,Muq,Mprop,Muvw,Umag,UeSP,dLCG,dmass,MdXi,Xg,Bb,Xb,Mb,Zg,Zb,Mvm,M_ext)
%Bx,Bv,Ba are the body motion position, velocity, acceleration in ship coordinate
%Wv,Wa are the wave particle velocity, acceleration in ship coordinate

u=Bv(1); v=Bv(2); w=Bv(3); p=Bv(4); q=Bv(5); r=Bv(6);
x=Bx(1); y=Bx(2); z=Bx(3); phi=Bx(4); theta=Bx(5); psi=Bx(6);
a1=Ba(1); a2=Ba(2); a3=Ba(3); a4=Ba(4); a5=Ba(5); a6=Ba(6); 

%MYuq=0.5*70.2^4*1025*Muq
%MYStat=Bb*9.81*dLCG*cos(theta)-Bb*9.81*(Zb-Zg)*sin(theta);

MYX1=0.5*70.2^3*1025*MdXi(1)*UeSP(1)^2;
MYX2=0.5*70.2^3*1025*MdXi(2)*UeSP(2)^2;
MYX3=0.5*70.2^3*1025*MdXi(3)*UeSP(3)^2;
MYX4=0.5*70.2^3*1025*MdXi(4)*UeSP(4)^2;
MYXb=0.5*70.2^3*1025*MdXi(5)*UeSP(5)^2;

MYApp_All=[MYX1; MYX2; MYX3; MYX4; MYXb;];

MYStat= BFM;
MYqq=0.5*70.2^5*1025*Mqq*q*abs(q);
MYuq=0.5*70.2^4*1025*u*q*1.9444E-03*1.1;

MYwq=0.5*70.2^4*1025*Mwq*w*abs(q);
MYuvw=0.5*70.2^3*1025*(Muvw)*Umag^2;
MYApp=(MYX1+MYX2+MYX3+MYX4+MYXb)*1;
Mprop=-1025*70.2^4*u*q*Mprop;

M_hull=MYuvw+MYuq;
MY_hyd=MYApp+MYStat+Mprop+M_hull;
MY=MYApp+MYStat+Mprop+M_hull+Mvm;
end

== matlab function ctrl_TT_ad_ctrl_cpp_ros_feedback/HDM/HDM B3/N/Mz ==
  data: Bx input; Bv input; Ba input; CNr input; CNrr input; CNvr input; CNuvw input; Umag input; UeX input; dLCG input; dmass input; CNdXi input; N output; NApp output; N_hull output; Xg parameter; Bb parameter; Xb parameter; Mb parameter; Zg parameter; Zb parameter; Nh_Total output; Nprop output; NStat output; Nvm input; BFN input
function [N,NApp,N_hull,Nh_Total,Nprop,NStat]  = fcn(Bx,Bv,Ba, CNr,CNrr,CNvr,CNuvw,Umag,UeX,dLCG,dmass,CNdXi,Xg,Bb,Xb,Mb,Zg,Zb,Nvm,BFN)
%Bx,Bv,Ba are the body motion position, velocity, acceleration in ship coordinate
%Wv,Wa are the wave particle velocity, acceleration in ship coordinate

u=Bv(1); v=Bv(2); w=Bv(3); p=Bv(4); q=Bv(5); r=Bv(6);
x=Bx(1); y=Bx(2); z=Bx(3); phi=Bx(4); theta=Bx(5); psi=Bx(6);
a1=Ba(1); a2=Ba(2); a3=Ba(3); a4=Ba(4); a5=Ba(5); a6=Ba(6); 

NdX1=70.2^3*1025*CNdXi(1)*UeX(1)^2;
NdX2=70.2^3*1025*CNdXi(2)*UeX(2)^2;
NdX3=70.2^3*1025*CNdXi(3)*UeX(3)^2;
NdX4=70.2^3*1025*CNdXi(4)*UeX(4)^2;

Nr  =0.5*70.2^3*1025*(7.6545E-03*0.8*u*r)*u^2*0.5;
%Nr  =-0.5*70.2^3*1025*CNr*u^2*3;
Nvr =0.5*70.2^3*1025*CNvr*u^2; %major source of error in it
Nrr =-0.5*70.2^3*1025*CNrr*r^2*u^2;
Nuvw=0.5*70.2^3*1025*CNuvw*Umag^2;
Nprop=0.5*70.2^3*1025*u^2*(-0.0055*r);

NApp=NdX1+NdX2+NdX3+NdX4;
N_hull=Nuvw+Nr+Nvr+Nrr;
NHullVM=N_hull+Nvm;
NStat= BFN;

Nh_Total=N_hull+NApp+NStat;

N=N_hull+NApp+NStat+Nvm;
end
